simulink library "FVT_lib"  (R2021b)
settings: Solver=VariableStepAuto  StartTime=0.0  StopTime=10.0  RelTol=1e-3
undefined symbols (not defined in the file): C_TASK_5MS_S, CANFDArray, ENUM_FAULTSTATE_FAIL, ENUM_FAULTSTATE_INDETERMINATE, ENUM_FAULTSTATE_PASS, EPSILON, FALSE, KHAL_CounterMAX_enum, KHAL_CounterMAXE2E_enum, LINArray, ONE_INT, TRUE, UNKNOWN, XX2KXX, ZERO_FLOAT, ZERO_INT
libraries: hdlsllib x41, simulink x24, hcu_lib x7
(part 1 of 3)
settings Model: Creator=user  LastModifiedBy=FVT23010
settings SolverCC: AlgebraicLoopSolver=TrustRegion
settings DebuggingCC: SFMachineParentedDataDiag=warning

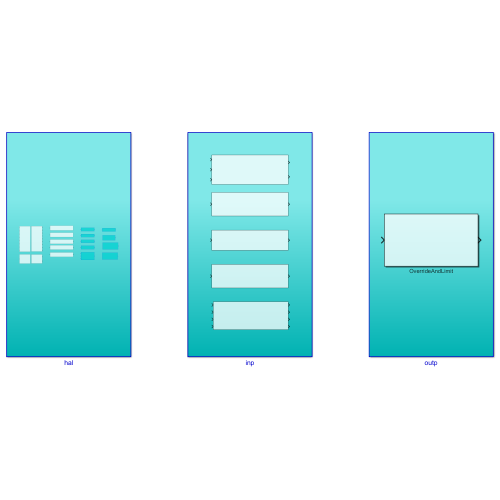
[thumbnail: Simulink's stored preview of the top-level diagram]
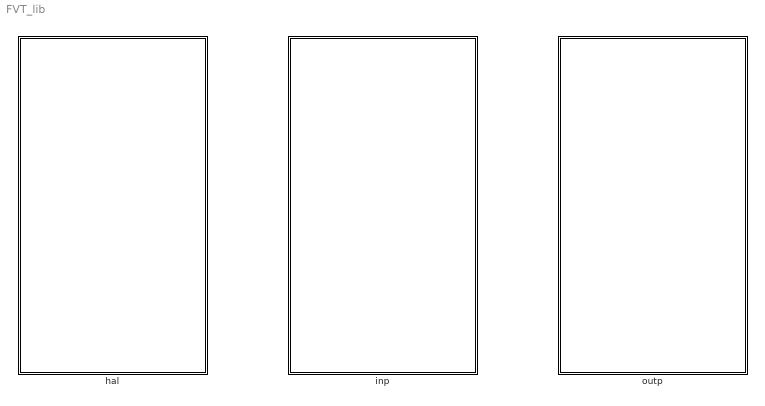
== system FVT_lib ==
  hal : Subsystem
  inp : Subsystem
  outp : Subsystem

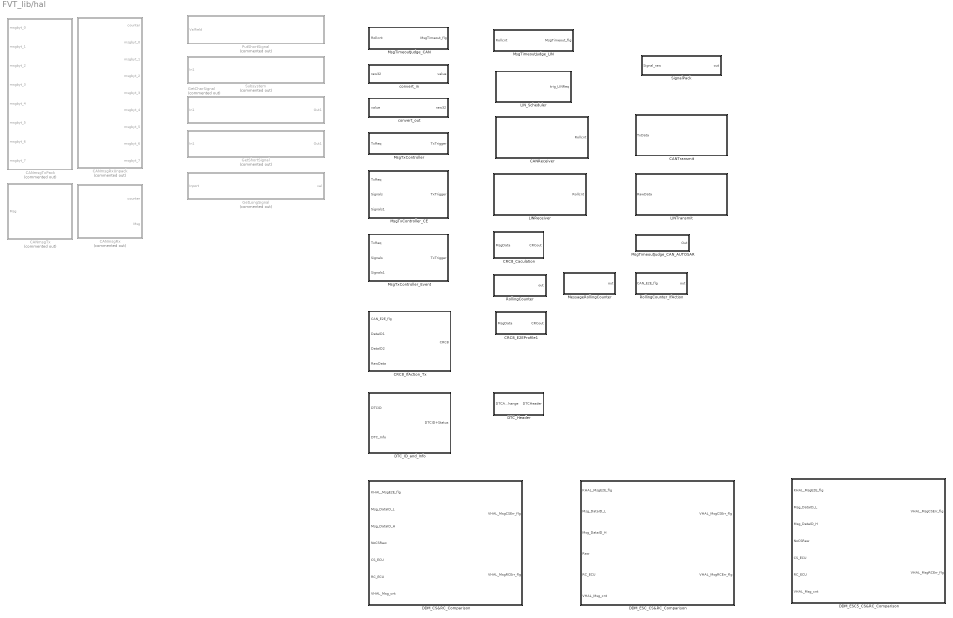
== system FVT_lib/hal ==
  CANReceiver : Subsystem  mask{busId=0, msgId=0x123, dlc=8}
      mask prompts: busId "BUS ID"; msgId "Message ID"
      mask Display:
      | fprintf('BUS ID: %1.0f \nMsg ID(hex): 0x%x \nDLC: %2.0f', busId, msgId,dlc);
      | 
      | port_label('output', 1, 'rolling counter');
  CANTransmit : Subsystem  mask{busId=0, msgId=0x123, dlc=8, IsCANFD=0}
      mask prompts: busId "BUS ID"; msgId "Message ID"
      mask Display:
      | fprintf('BUS ID: %1.0f \nMsg ID(hex): 0x%x \nDLC: %2.0f\nIs CANFD: %1.0f', busId, msgId,dlc,IsCANFD);
      | port_label('input', 1, 'Tx raw data');
  CANmsgRx : Subsystem  Commented=on  mask{rtwchn=CAN 1, rtwcode=367}
      mask prompts: rtwchn "Can channel :"; rtwcode "CAN ID :"
      mask TypeOptions rtwchn: CAN 1 | CAN 2 | CAN 3 | CAN 4
      mask Display:
      | fprintf('Receive Message on\nCAN %x \nID_hex: %x', rtwchn, rtwcode);
      | image('nxp_logo.png','top-left')
      | port_label('output', 1, 'rolling counter');
  CANmsgRxUnpack : Subsystem  Commented=on  mask{rtwchn=CAN 1, rtwcode=367}
      mask prompts: rtwchn "Can channel :"; rtwcode "CAN ID :"
      mask TypeOptions rtwchn: CAN 1 | CAN 2 | CAN 3 | CAN 4
      mask Display:
      | fprintf('Receive Message on\nCAN %x \nID_hex: %x', rtwchn, rtwcode);
      | image('nxp_logo.png','top-left')
      | port_label('output', 1, 'rolling counter');
  CANmsgTx : Subsystem  Commented=on  mask{rtwchn=CAN 1, rtwmrk=FALSE, rtwcode=367}
      mask prompts: rtwchn "Can channel :"; rtwmrk "Extend ID :"; rtwcode "CAN ID :"
      mask TypeOptions rtwchn: CAN 1 | CAN 2 | CAN 3 | CAN 4
      mask TypeOptions rtwmrk: FALSE | TRUE
      mask Display:
      | fprintf('Send Message on\nCAN %x \nID_hex: %x', rtwchn, rtwcode);
      | image('nxp_logo.png','top-left')
  CANmsgTxPack : Subsystem  Commented=on  mask{rtwchn=CAN 1, rtwmrk=FALSE, rtwcode=367}
      mask prompts: rtwchn "Can channel :"; rtwmrk "Extend ID :"; rtwcode "CAN ID :"
      mask TypeOptions rtwchn: CAN 1 | CAN 2 | CAN 3 | CAN 4
      mask TypeOptions rtwmrk: FALSE | TRUE
      mask Display:
      | fprintf('Send Message on\nCAN %x \nID_hex: %x', rtwchn, rtwcode);
      | image('nxp_logo.png','top-left')
  CRC8_Caculation : Subsystem
      mask help: MeasumentTrigerEvent
      mask Display: fprintf('CRC8');
  CRC8_E2EProfile1 : Subsystem
      mask help: MeasumentTrigerEvent
      mask Display: fprintf('CRC8_E2EProfile1');
  CRC8_IfAction_Tx : Subsystem
      mask help: MeasumentTrigerEvent
      mask Display: fprintf('CRC8_IfAction');
  DDM_CS&RC_Comparison : Subsystem  mask{MsgCycleTime=0}
      mask help: CS&RC Comparison
      mask Display:
      | fprintf('DDM_CS&RC_Comparison');
      | 
      | port_label('input', 1, 'KHAL_MsgE2E_flg');
      | port_label('input', 2, 'Msg_DataID_L');
      | port_label('input', 3, 'Msg_DataID_H');
      | port_label('input', 4, 'NoCSRaw');
      | port_label('input', 5, 'CS_ECU');
      | port_label('input', 6, 'RC_ECU');
      | port_label('input', 7, 'VHAL_Msg_cnt');
      | 
      | port_label('output', 1, 'VHAL_MsgCSErr_flg');
      | port_label('output', 2, 'VHAL_MsgRCErr_flg');
  DDM_ESC5_CS&RC_Comparison : Subsystem  mask{MsgCycleTime=0}
      mask help: CS&RC Comparison
      mask Display:
      | fprintf('DDM_ESC5_CS&RC_Comparison');
      | 
      | port_label('input', 1, 'KHAL_MsgE2E_flg');
      | port_label('input', 2, 'Msg_DataID_L');
      | port_label('input', 3, 'Msg_DataID_H');
      | port_label('input', 4, 'NoCSRaw');
      | port_label('input', 5, 'CS_ECU');
      | port_label('input', 6, 'RC_ECU');
      | port_label('input', 7, 'VHAL_Msg_cnt');
      | 
      | port_label('output', 1, 'VHAL_MsgCSErr_flg');
      | port_label('output', 2, 'VHAL_MsgRCErr_flg');
  DDM_ESC_CS&RC_Comparison : Subsystem  mask{MsgCycleTime=0}
      mask help: CS&RC Comparison
      mask Display:
      | fprintf('DDM_ESC_CS&RC_Comparison');
      | 
      | port_label('input', 1, 'KHAL_MsgE2E_flg');
      | port_label('input', 2, 'Msg_DataID_L');
      | port_label('input', 3, 'Msg_DataID_H');
      | port_label('input', 4, 'Raw');
      | port_label('input', 5, 'RC_ECU');
      | port_label('input', 6, 'VHAL_Msg_cnt');
      | 
      | port_label('output', 1, 'VHAL_MsgCSErr_flg');
      | port_label('output', 2, 'VHAL_MsgRCErr_flg');
  DTC_Header : Subsystem
      mask help: MeasumentTrigerEvent
      mask Display: fprintf('DTCHeader');
  DTC_ID_and_Info : Subsystem
      mask help: MeasumentTrigerEvent
      mask Display: fprintf('DTCID+Info');
  GetCharSignal : Subsystem  Commented=on  mask{CC1=55, CC2=8}
      mask prompts: CC1 "MSB:"; CC2 "DataLegth:"
      mask TypeOptions CC1: 0 | 1 | 2 | 3 | 4 | 5 | 6 | 7 | 8 | 9 | 10 | 11 | 12 | 13 | 14 | 15 | 16 | 17 | 18 | 19 | 20 | 21 | 22 | 23 | 24 | 25 | 26 | 27 | 28 | 29 | 30 | 31 | 32 | 33 | 34 | 35 | 36 | 37 | 38 | 39 | 40 | 41 | 42 | 43 | 44 | 45 | 46 | 47 | 48 | 49 | 50 | 51 | 52 | 53 | 54 | 55 | 56 | 57 | 58 | 59 | 60 | 61 | 62 | 63
      mask Display:
      | fprintf('Get Char Signal \nMSB: %d \nDLC: %d', CC1-1, CC2);
      | image('nxp_logo.png','top-left')
  GetLongSignal : Subsystem  Commented=on  mask{msb=0, len=0}
      mask prompts: len "Length"
      mask Display:
      | fprintf('Get Long Signal \nMSB: %d \nDLC: %d', msb, len);
      | image('nxp_logo.png','top-left')
  GetShortSignal : Subsystem  Commented=on  mask{CC1=23, CC2=12}
      mask prompts: CC1 "MSB:"; CC2 "DataLegth:"
      mask TypeOptions CC1: 0 | 1 | 2 | 3 | 4 | 5 | 6 | 7 | 8 | 9 | 10 | 11 | 12 | 13 | 14 | 15 | 16 | 17 | 18 | 19 | 20 | 21 | 22 | 23 | 24 | 25 | 26 | 27 | 28 | 29 | 30 | 31 | 32 | 33 | 34 | 35 | 36 | 37 | 38 | 39 | 40 | 41 | 42 | 43 | 44 | 45 | 46 | 47 | 48 | 49 | 50 | 51 | 52 | 53 | 54 | 55 | 56 | 57 | 58 | 59 | 60 | 61 | 62 | 63
      mask Display:
      | fprintf('Get Short Signal \nMSB: %d \nDLC: %d', CC1-1, CC2);
      | image('nxp_logo.png','top-left')
  LINReceiver : Subsystem  mask{busId=0, msgId=0x123, dlc=8}
      mask prompts: busId "BUS ID"; msgId "Message ID"
      mask Display:
      | fprintf('BUS ID: %1.0f \nMsg ID(hex): 0x%x \nDLC: %2.0f', busId, msgId,dlc);
      | port_label('output', 1, 'fault counter');
  LINTransmit : Subsystem  mask{busId=0, msgId=0x123, dlc=8}
      mask prompts: busId "BUS ID"; msgId "Message ID"
      mask Display:
      | fprintf('BUS ID: %1.0f \nMsg ID(hex): 0x%x \nDLC: %2.0f', busId, msgId,dlc);
      | port_label('input', 1, 'Tx raw data');
  LIN_Scheduler : Subsystem  mask{CycleTime=100, FirstDelayTime=80}
      mask prompts: CycleTime "CycleTime_ms"; FirstDelayTime "DelayTime_ms"
      mask Display: fprintf('Total cycle time(ms): %d\nFirst delay time(ms): %3.0f', CycleTime, FirstDelayTime);
  MessageRollingCounter : Subsystem  mask{CounterMAX=14, task_time_ms=5, msg_time_ms=10}
      mask help: MeasumentTrigerEvent
      mask Display: fprintf('MsgRC');
  MsgTimeoutJudge_CAN : Subsystem  mask{Gain=1.5, CycleTime=100}
      mask prompts: CycleTime "MsgCycleTime_ms"
      mask help: MeasumentTrigerTime
      mask Display: fprintf('Gain: %4.2f \nMsg Cycletime ms: %3.0f', Gain, CycleTime);
  MsgTimeoutJudge_CAN_AUTOSAR : Subsystem
      mask help: MeasumentTrigerEvent
      mask Display: fprintf('MsgTimeoutJudge_CAN\nAUTOSAR');
  MsgTimeoutJudge_LIN : Subsystem  mask{TimeoutCnt=3}
      mask help: MeasumentTrigerTime
      mask Display: fprintf('TimeoutCnt: %4.2f', TimeoutCnt);
  MsgTxController : Subsystem  mask{CycleTime=100}
      mask prompts: CycleTime "MsgCycleTime_ms"
      mask help: MeasumentTrigerTime
      mask Display: fprintf('Tx Method: Cycle\nMsg Cycletime ms: %3.0f', CycleTime);
  MsgTxController_CE : Subsystem  mask{CycleTime=100}
      mask prompts: CycleTime "MsgCycleTime_ms"
      mask help: MeasumentTrigerTime
      mask Display: fprintf('Tx Method: CE\nMsg Cycletime ms: %3.0f', CycleTime);
  MsgTxController_Event : Subsystem
      mask help: MeasumentTrigerEvent
      mask Display: fprintf('Tx Method: Event');
  PutShortSignal : Subsystem  Commented=on  mask{SS1=5, SS2=13, SS3=[0 0 0 0 0 0 0 0]}
      mask prompts: SS1 "MSB:"; SS2 "DataLeght:"; SS3 "MsgBuffer:"
      mask TypeOptions SS1: 0 | 1 | 2 | 3 | 4 | 5 | 6 | 7 | 8 | 9 | 10 | 11 | 12 | 13 | 14 | 15 | 16 | 17 | 18 | 19 | 20 | 21 | 22 | 23 | 24 | 25 | 26 | 27 | 28 | 29 | 30 | 31 | 32 | 33 | 34 | 35 | 36 | 37 | 38 | 39 | 40 | 41 | 42 | 43 | 44 | 45 | 46 | 47 | 48 | 49 | 50 | 51 | 52 | 53 | 54 | 55 | 56 | 57 | 58 | 59 | 60 | 61 | 62 | 63
      mask Display:
      | fprintf('Put Short Signal \nMSB: %d \nDLC: %d', SS1-1, SS2);
      | image('nxp_logo.png','top-left')
  RollingCounter : Subsystem  mask{CounterMAX=14}
      mask help: MeasumentTrigerEvent
      mask Display: fprintf('RollingCounter');
  RollingCounter_IfAction : Subsystem
      mask help: MeasumentTrigerEvent
      mask Display: fprintf('RollingCounter_IfAction');
  SignalPack : Subsystem  mask(ConvertOut){RightShiftCnt=0, BitMask=2^1-1, LeftShiftCnt=0}
      mask prompts: BitMask "Bit mask"
      mask help:
      | Conversion Formula
      |
      | The conversion formula is
      |
      | raw_value = (physical_value - Offset) / Factor
      |
      | where physical_value is the value of the signal after it is saturated using the specified Min and Max values. raw_value is the packed signal value.
      mask Display: fprintf('RightShiftCnt: %1.0f \nMASK: %d \nLeftShiftCnt: %1.0f', RightShiftCnt, BitMask, LeftShiftCnt);
  Subsystem : Subsystem  Commented=on  mask{SS1=47, SS2=8, SS3=[0 0 0 0 0 0 0 0]}
      mask prompts: SS1 "MSB:"; SS2 "DataLegth:"; SS3 "MsgBuffer:"
      mask TypeOptions SS1: 0 | 1 | 2 | 3 | 4 | 5 | 6 | 7 | 8 | 9 | 10 | 11 | 12 | 13 | 14 | 15 | 16 | 17 | 18 | 19 | 20 | 21 | 22 | 23 | 24 | 25 | 26 | 27 | 28 | 29 | 30 | 31 | 32 | 33 | 34 | 35 | 36 | 37 | 38 | 39 | 40 | 41 | 42 | 43 | 44 | 45 | 46 | 47 | 48 | 49 | 50 | 51 | 52 | 53 | 54 | 55 | 56 | 57 | 58 | 59 | 60 | 61 | 62 | 63
      mask Display:
      | fprintf('Put Char Signal \nMSB: %d \nDLC: %d', SS1-1, SS2);
      | image('nxp_logo.png','top-left')
  convert_in : Subsystem  mask(ConvertIn){gain=1, offset=1}
      mask help:
      | Conversion Formula
      |
      | The conversion formula is
      |
      | raw_value = (physical_value - Offset) / Factor
      |
      | where physical_value is the value of the signal after it is saturated using the specified Min and Max values. raw_value is the packed signal value.
      mask Display: fprintf('Resolution: %6.4f \nOffset: %5.0f', gain, offset);
  convert_out : Subsystem  mask(ConvertOut){gain=1, offset=1}
      mask help:
      | Conversion Formula
      |
      | The conversion formula is
      |
      | raw_value = (physical_value - Offset) / Factor
      |
      | where physical_value is the value of the signal after it is saturated using the specified Min and Max values. raw_value is the packed signal value.
      mask Display: fprintf('Resolution: %6.4f \nOffset: %5.0f', gain, offset);

== system FVT_lib/inp ==
  CAN_Msg_Validity_Process_template : Subsystem
  ad_signal_template : Subsystem
  can_signal_template : Subsystem
      settings: RTWSystemCode=Inline
  di_signal_template : Subsystem
  pwm_signal_template : Subsystem

== system FVT_lib/outp ==
  OverrideAndLimit : Subsystem

== system FVT_lib/hal/CANReceiver ==
  CANReceive : CCaller  FunctionName=CANReceive  PortSpecificationStruct="%)30     .    T @   8    (     @         %    \"     4    !     0         %  0 \"0    $    _    07)G3F%M90  4&]R=$YA;64 4V-O<&4     26YD97@     5'EP90      4VEZ90      27-';&]B86P   X    P    !@    @    $          4    (     0    ,    !         !   P!O=70 #@   #     &    \"     0         !0    @    !     P    $         $  # &]U=  .    .     8    (    !          %    \"     $    &     0         0   ...(+2654 chars)"
  Constant6 : Constant  Value=busId
  Constant7 : Constant  Value=CANFDArray
  Constant8 : Constant  Value=msgId
  Constant9 : Constant  Value=dlc
  Data Type Conversion16 : DataTypeConversion  OutDataTypeStr=uint8
  Data Type Conversion17 : DataTypeConversion  OutDataTypeStr=uint16
  Data Type Conversion18 : DataTypeConversion  OutDataTypeStr=uint8
  Data Type Conversion19 : DataTypeConversion  OutDataTypeStr=uint8
  Demux : Demux  Outputs=16
  Rollcnt : Outport
  wires:
  Data Type Conversion19/1 -> CANReceive/3
  Constant8/1 -> Data Type Conversion17/1
  Constant6/1 -> Data Type Conversion16/1
  Constant9/1 -> Data Type Conversion18/1
  Data Type Conversion17/1 -> CANReceive/2
  Data Type Conversion16/1 -> CANReceive/1
  Data Type Conversion18/1 -> CANReceive/4
  Constant7/1 -> Data Type Conversion19/1
  [RxData] -> Demux/1
  CANReceive/2 -> [RxData]
  CANReceive/1 -> Rollcnt/1

== system FVT_lib/hal/CANTransmit ==
  TxData : Inport
  C Caller : CCaller  FunctionName=CANTransmit  PortSpecificationStruct="%)30     .    R @   8    (     @         %    \"     4    !     0         %  0 \"0    $    _    07)G3F%M90  4&]R=$YA;64 4V-O<&4     26YD97@     5'EP90      4VEZ90      27-';&]B86P   X    X    !@    @    $          4    (     0    4    !         !     %    8G5S260    .    .     8    (    !          %    \"     $    %     0         0    !0   &)U<TED    #@   #@    &    \"     0         !0    @    !   ...(+2646 chars)"
  Constant2 : Constant  Value=busId
  Constant3 : Constant  Value=msgId
  Constant4 : Constant  Value=IsCANFD
  Constant5 : Constant  Value=dlc
  UnitConverter5 : DataTypeConversion  OutDataTypeStr=uint8
  UnitConverter6 : DataTypeConversion  OutDataTypeStr=uint16
  UnitConverter7 : DataTypeConversion  OutDataTypeStr=uint8
  UnitConverter8 : DataTypeConversion  OutDataTypeStr=uint8
  wires:
  UnitConverter7/1 -> C Caller/3
  UnitConverter6/1 -> C Caller/2
  UnitConverter5/1 -> C Caller/1
  Constant5/1 -> UnitConverter8/1
  Constant3/1 -> UnitConverter6/1
  Constant4/1 -> UnitConverter7/1
  Constant2/1 -> UnitConverter5/1
  UnitConverter8/1 -> C Caller/5
  TxData/1 -> C Caller/4

== system FVT_lib/hal/CANmsgRx ==
  Constant : Constant  Value=rtwcode  OutDataTypeStr=uint32
  Data Type Conversion7 : DataTypeConversion  OutDataTypeStr=uint8
  sfcnCanLLGetMessage : S-Function  FunctionName=sfcnCanLLGetMessage  Parameters=SParameter1  SFunctionDeploymentMode=off  EnableBusSupport=off  mask{SParameter1=rtwchn-1}
      mask prompts: SParameter1 "P1:"
      mask Display: fprintf('Level-2 S-Function CanLLGetMessage');
  counter : Outport
  Msg : Outport  Port=2
  wires:
  Data Type Conversion7/1 -> counter/1
  sfcnCanLLGetMessage/1 -> Data Type Conversion7/1
  Constant/1 -> sfcnCanLLGetMessage/1
  sfcnCanLLGetMessage/2 -> Msg/1

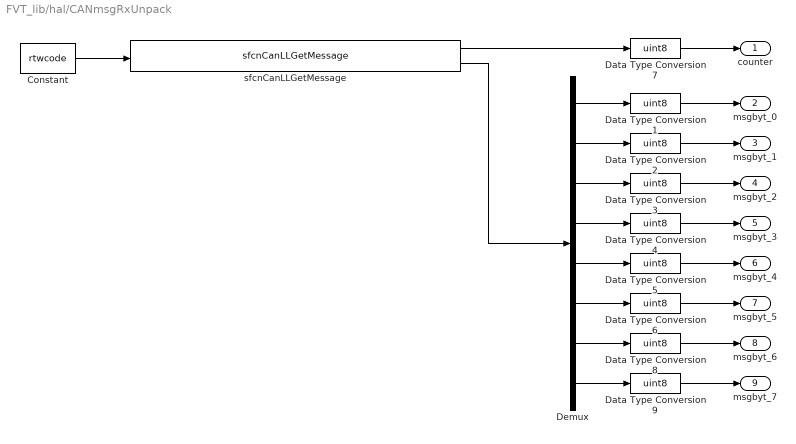
== system FVT_lib/hal/CANmsgRxUnpack ==
  Constant : Constant  Value=rtwcode  OutDataTypeStr=uint32
  Data Type Conversion{1..9} (9 alike) : DataTypeConversion  OutDataTypeStr=uint8
  Demux : Demux  Outputs=8
  sfcnCanLLGetMessage : S-Function  FunctionName=sfcnCanLLGetMessage  Parameters=SParameter1  SFunctionDeploymentMode=off  EnableBusSupport=off  mask{SParameter1=rtwchn-1}
      mask prompts: SParameter1 "P1:"
      mask Display: fprintf('Level-2 S-Function CanLLGetMessage');
  counter : Outport
  msgbyt_0 : Outport  Port=2
  msgbyt_1 : Outport  Port=3
  msgbyt_2 : Outport  Port=4
  msgbyt_3 : Outport  Port=5
  msgbyt_4 : Outport  Port=6
  msgbyt_5 : Outport  Port=7
  msgbyt_6 : Outport  Port=8
  msgbyt_7 : Outport  Port=9
  wires:
  Demux/1 -> Data Type Conversion1/1
  Demux/4 -> Data Type Conversion4/1
  Constant/1 -> sfcnCanLLGetMessage/1
  Demux/6 -> Data Type Conversion6/1
  Demux/3 -> Data Type Conversion3/1
  Demux/8 -> Data Type Conversion9/1
  Demux/2 -> Data Type Conversion2/1
  Demux/5 -> Data Type Conversion5/1
  Demux/7 -> Data Type Conversion8/1
  sfcnCanLLGetMessage/1 -> Data Type Conversion7/1
  sfcnCanLLGetMessage/2 -> Demux/1
  Data Type Conversion7/1 -> counter/1
  Data Type Conversion1/1 -> msgbyt_0/1
  Data Type Conversion2/1 -> msgbyt_1/1
  Data Type Conversion4/1 -> msgbyt_3/1
  Data Type Conversion3/1 -> msgbyt_2/1
  Data Type Conversion5/1 -> msgbyt_4/1
  Data Type Conversion8/1 -> msgbyt_6/1
  Data Type Conversion6/1 -> msgbyt_5/1
  Data Type Conversion9/1 -> msgbyt_7/1

== system FVT_lib/hal/CANmsgTx ==
  Msg : Inport
  Constant4 : Constant  Value=rtwcode  OutDataTypeStr=uint32
  Constant6 : Constant  Value=rtwmrk-1  OutDataTypeStr=uint8
  Data Type Conversion : DataTypeConversion  OutDataTypeStr=uint8
  sfcnCanLLSendMessage : S-Function  FunctionName=sfcnCanLLSendMessage  Parameters=SParameter1  SFunctionDeploymentMode=off  EnableBusSupport=off  mask{SParameter1=rtwchn-1}
      mask prompts: SParameter1 "P1:"
      mask Display: fprintf('Level-2 S-Function CanLLSendMessage');
  wires:
  Data Type Conversion/1 -> sfcnCanLLSendMessage/3
  Msg/1 -> Data Type Conversion/1
  Constant4/1 -> sfcnCanLLSendMessage/1
  Constant6/1 -> sfcnCanLLSendMessage/2

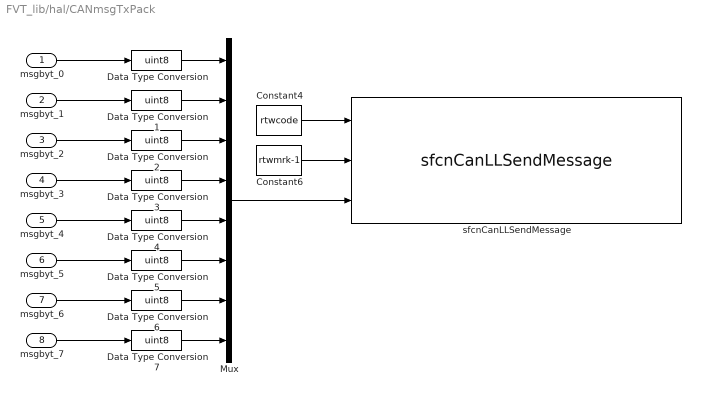
== system FVT_lib/hal/CANmsgTxPack ==
  msgbyt_0 : Inport
  msgbyt_1 : Inport  Port=2
  msgbyt_2 : Inport  Port=3
  msgbyt_3 : Inport  Port=4
  msgbyt_4 : Inport  Port=5
  msgbyt_5 : Inport  Port=6
  msgbyt_6 : Inport  Port=7
  msgbyt_7 : Inport  Port=8
  Constant4 : Constant  Value=rtwcode  OutDataTypeStr=uint32
  Constant6 : Constant  Value=rtwmrk-1  OutDataTypeStr=uint8
  Data Type Conversion{,1..7} (8 alike) : DataTypeConversion  OutDataTypeStr=uint8
  Mux : Mux  Inputs=8
  sfcnCanLLSendMessage : S-Function  FunctionName=sfcnCanLLSendMessage  Parameters=SParameter1  SFunctionDeploymentMode=off  EnableBusSupport=off  mask{SParameter1=rtwchn-1}
      mask prompts: SParameter1 "P1:"
      mask Display: fprintf('Level-2 S-Function CanLLSendMessage');
  wires:
  Constant6/1 -> sfcnCanLLSendMessage/2
  Constant4/1 -> sfcnCanLLSendMessage/1
  msgbyt_1/1 -> Data Type Conversion1/1
  msgbyt_3/1 -> Data Type Conversion3/1
  msgbyt_6/1 -> Data Type Conversion6/1
  msgbyt_5/1 -> Data Type Conversion5/1
  msgbyt_0/1 -> Data Type Conversion/1
  msgbyt_7/1 -> Data Type Conversion7/1
  msgbyt_4/1 -> Data Type Conversion4/1
  msgbyt_2/1 -> Data Type Conversion2/1
  Mux/1 -> sfcnCanLLSendMessage/3
  Data Type Conversion/1 -> Mux/1
  Data Type Conversion1/1 -> Mux/2
  Data Type Conversion2/1 -> Mux/3
  Data Type Conversion3/1 -> Mux/4
  Data Type Conversion4/1 -> Mux/5
  Data Type Conversion5/1 -> Mux/6
  Data Type Conversion6/1 -> Mux/7
  Data Type Conversion7/1 -> Mux/8

== system FVT_lib/hal/CRC8_Caculation ==
  MsgData : Inport
  Data Type Conversion3 : DataTypeConversion  OutDataTypeStr=uint8
  Data Type Conversion4 : DataTypeConversion  OutDataTypeStr=uint8
  MATLAB Function : MATLAB Function  TreatAsAtomicUnit=on
  CRCout : Outport
  wires:
  Data Type Conversion4/1 -> CRCout/1
  MATLAB Function/1(CRC_Out) -> Data Type Conversion4/1
  Data Type Conversion3/1 -> MATLAB Function/1(msg_raw)
  MsgData/1 -> Data Type Conversion3/1

== system FVT_lib/hal/CRC8_E2EProfile1 ==
  MsgData : Inport
  Data Type Conversion3 : DataTypeConversion  OutDataTypeStr=uint8
  Data Type Conversion4 : DataTypeConversion  OutDataTypeStr=uint8
  MATLAB Function : MATLAB Function  TreatAsAtomicUnit=on
  CRCout : Outport
  wires:
  MsgData/1 -> Data Type Conversion3/1
  Data Type Conversion3/1 -> MATLAB Function/1(msg_raw)
  MATLAB Function/1(CRC_Out) -> Data Type Conversion4/1
  Data Type Conversion4/1 -> CRCout/1

== system FVT_lib/hal/CRC8_IfAction_Tx ==
  CAN_E2E_flg : Inport
  DataID1 : Inport  Port=2
  DataID2 : Inport  Port=3
  RawData : Inport  Port=4
  Data Type Conversion : DataTypeConversion  OutDataTypeStr=uint8
  If : If
  If Action Subsystem : Subsystem  TreatAsAtomicUnit=on
  If Action Subsystem1 : Subsystem  TreatAsAtomicUnit=on
  Merge : Merge
  CRC8 : Outport
  wires:
  Data Type Conversion/1 -> If/1
  Merge/1 -> CRC8/1
  If Action Subsystem/1(CRC8_Result) -> Merge/2
  If Action Subsystem1/1(CRC8_E2EResult) -> Merge/1
  [RawData] -> If Action Subsystem/1(Byte1)
  [RawData] -> If Action Subsystem1/3(Byte1)
  [DataID2] -> If Action Subsystem1/2(CAN_E2E_ID2)
  [DataID1] -> If Action Subsystem1/1(CAN_E2E_ID1)
  [CAN_E2E_flg] -> Data Type Conversion/1
  RawData/1 -> [RawData]
  DataID2/1 -> [DataID2]
  DataID1/1 -> [DataID1]
  CAN_E2E_flg/1 -> [CAN_E2E_flg]
  If/1 -> If Action Subsystem1/Action
  If/2 -> If Action Subsystem/Action

== system FVT_lib/hal/DDM_CS&RC_Comparison ==
  KHAL_MsgE2E_flg : Inport
  Msg_DataID_L : Inport  Port=2
  Msg_DataID_H : Inport  Port=3
  NoCSRaw : Inport  Port=4
  CS_ECU : Inport  Port=5
  RC_ECU : Inport  Port=6
  VHAL_Msg_cnt : Inport  Port=7
  CRC8_Compare : Subsystem  mask{MissingNumLimit=2, RepeatNumLimit=1, CounterMAX=15, CounterMAX_E2E=14}
      mask help: MeasumentTrigerEvent
      mask Display: fprintf('CS & RC_Compare');
  CRC8_IfAction_Rx : Subsystem
      mask help: MeasumentTrigerEvent
      mask Display: fprintf('CRC8_IfAction');
  Constant5 : Constant  Value=MsgCycleTime  OutDataTypeStr=single
  Gain : Gain  Gain=1.5
  Gain1 : Gain  Gain=XX2KXX
  VHAL_MsgCSErr_flg : Outport
  VHAL_MsgRCErr_flg : Outport  Port=2
  wires:
  Msg_DataID_H/1 -> CRC8_IfAction_Rx/3(CAN_E2E_ID2)
  Msg_DataID_L/1 -> CRC8_IfAction_Rx/2(CAN_E2E_ID1)
  KHAL_MsgE2E_flg/1 -> CRC8_Compare/5(CAN_E2E_flg), CRC8_IfAction_Rx/1(CAN_E2E_flg)
  CRC8_Compare/1(CS_Error) -> VHAL_MsgCSErr_flg/1
  CRC8_Compare/2(RC_Error) -> VHAL_MsgRCErr_flg/1
  CS_ECU/1 -> CRC8_Compare/1(MsgData)
  NoCSRaw/1 -> CRC8_Compare/6(noCSRaw), CRC8_IfAction_Rx/4(Raw)
  RC_ECU/1 -> CRC8_Compare/3(RC)
  VHAL_Msg_cnt/1 -> CRC8_Compare/4(MsgCnt)
  CRC8_IfAction_Rx/1(CRC8) -> CRC8_Compare/2(CRC8_Data)
  Gain/1 -> CRC8_Compare/7(RepeatTimeLimit)
  Constant5/1 -> Gain1/1
  Gain1/1 -> Gain/1

== system FVT_lib/hal/DDM_ESC5_CS&RC_Comparison ==
  KHAL_MsgE2E_flg : Inport
  Msg_DataID_L : Inport  Port=2
  Msg_DataID_H : Inport  Port=3
  NoCSRaw : Inport  Port=4
  CS_ECU : Inport  Port=5
  RC_ECU : Inport  Port=6
  VHAL_Msg_cnt : Inport  Port=7
  CRC8_Compare : Subsystem  mask{MissingNumLimit=2, RepeatNumLimit=1, CounterMAX=15, CounterMAX_E2E=14}
      mask help: MeasumentTrigerEvent
      mask Display: fprintf('CS & RC_Compare');
  CRC8_IfAction_Rx : Subsystem
      mask help: MeasumentTrigerEvent
      mask Display: fprintf('CRC8_IfAction');
  Constant5 : Constant  Value=MsgCycleTime  OutDataTypeStr=single
  Gain : Gain  Gain=1.5
  Gain1 : Gain  Gain=XX2KXX
  VHAL_MsgCSErr_flg : Outport
  VHAL_MsgRCErr_flg : Outport  Port=2
  wires:
  CRC8_IfAction_Rx/1(CRC8) -> CRC8_Compare/2(CRC8_Data)
  VHAL_Msg_cnt/1 -> CRC8_Compare/4(MsgCnt)
  RC_ECU/1 -> CRC8_Compare/3(RC)
  NoCSRaw/1 -> CRC8_Compare/6(noCSRaw), CRC8_IfAction_Rx/4(Raw)
  CS_ECU/1 -> CRC8_Compare/1(MsgData)
  CRC8_Compare/2(RC_Error) -> VHAL_MsgRCErr_flg/1
  CRC8_Compare/1(CS_Error) -> VHAL_MsgCSErr_flg/1
  KHAL_MsgE2E_flg/1 -> CRC8_IfAction_Rx/1(CAN_E2E_flg), CRC8_Compare/5(CAN_E2E_flg)
  Msg_DataID_L/1 -> CRC8_IfAction_Rx/2(CAN_E2E_ID1)
  Msg_DataID_H/1 -> CRC8_IfAction_Rx/3(CAN_E2E_ID2)
  Constant5/1 -> Gain1/1
  Gain/1 -> CRC8_Compare/7(RepeatTimeLimit)
  Gain1/1 -> Gain/1

== system FVT_lib/hal/DDM_ESC_CS&RC_Comparison ==
  KHAL_MsgE2E_flg : Inport
  Msg_DataID_L : Inport  Port=2
  Msg_DataID_H : Inport  Port=3
  Raw : Inport  Port=4
  RC_ECU : Inport  Port=5
  VHAL_Msg_cnt : Inport  Port=6
  Constant5 : Constant  Value=MsgCycleTime  OutDataTypeStr=single
  Demux : Demux  Outputs=8
  ESC_CS_Comparison : Subsystem
      mask help: ESC CS Comparison
      mask Display:
      | fprintf('ESC_CS_Comparison');
      | 
      | port_label('input', 1, 'Byte0');
      | port_label('input', 2, 'Byte1');
      | port_label('input', 3, 'Byte2');
      | port_label('input', 4, 'Byte3');
      | port_label('input', 5, 'Byte4');
      | port_label('input', 6, 'Byte5');
      | port_label('input', 7, 'Byte6');
      | port_label('input', 8, 'Byte7');
      | 
      | port_label('output', 1, 'CS_Equal_flg');
  Gain : Gain  Gain=1.5
  Gain1 : Gain  Gain=XX2KXX
  Logical Operator : Logic  Operator=NOT  AllPortsSameDT=off  OutDataTypeStr=boolean
  RC_Compare : Subsystem  mask{MissingNumLimit=2, RepeatNumLimit=1, CounterMAX=15, CounterMAX_E2E=14}
      mask help: MeasumentTrigerEvent
      mask Display: fprintf('RC_Compare');
  Terminator : Terminator
  Terminator1 : Terminator
  VHAL_MsgCSErr_flg : Outport
  VHAL_MsgRCErr_flg : Outport  Port=2
  wires:
  VHAL_Msg_cnt/1 -> RC_Compare/2(MsgCnt)
  RC_ECU/1 -> RC_Compare/1(RC)
  RC_Compare/1(RC_Error) -> VHAL_MsgRCErr_flg/1
  ESC_CS_Comparison/1(CS_Equal_flg) -> Logical Operator/1
  Logical Operator/1 -> VHAL_MsgCSErr_flg/1
  KHAL_MsgE2E_flg/1 -> RC_Compare/3(CAN_E2E_flg)
  Demux/1 -> ESC_CS_Comparison/1(byte0)
  Demux/2 -> ESC_CS_Comparison/2(byte1)
  Demux/3 -> ESC_CS_Comparison/3(byte2)
  Demux/4 -> ESC_CS_Comparison/4(byte3)
  Demux/5 -> ESC_CS_Comparison/5(byte4)
  Demux/6 -> ESC_CS_Comparison/6(byte5)
  Demux/7 -> ESC_CS_Comparison/7(byte6)
  Demux/8 -> ESC_CS_Comparison/8(byte7)
  Raw/1 -> RC_Compare/4(noCSRaw), Demux/1
  Msg_DataID_L/1 -> Terminator/1
  Msg_DataID_H/1 -> Terminator1/1
  Constant5/1 -> Gain1/1
  Gain/1 -> RC_Compare/5(RepeatTimeLimit)
  Gain1/1 -> Gain/1

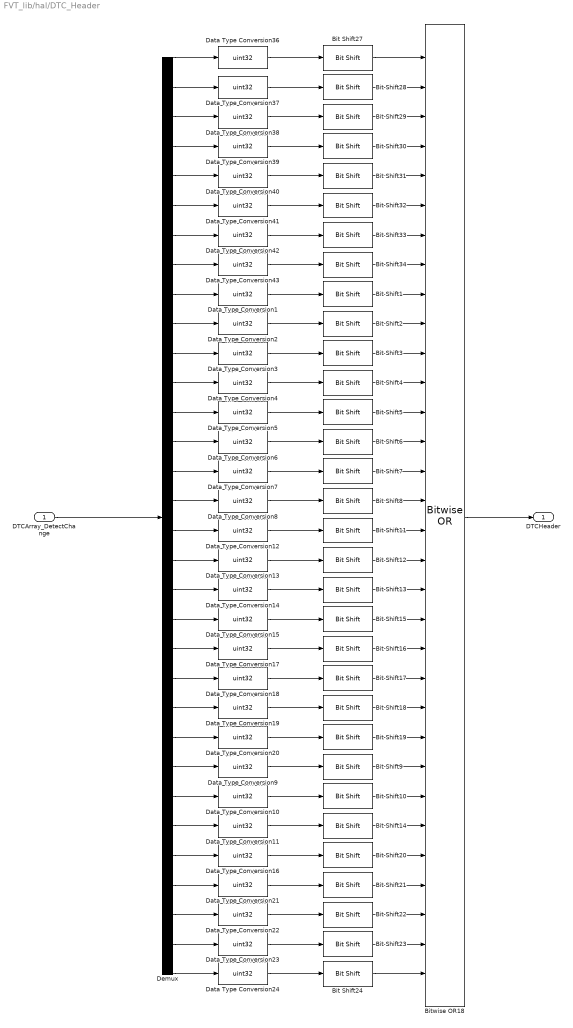
== system FVT_lib/hal/DTC_Header ==
  DTCArray_DetectChange : Inport
  Bit Shift1 : hdlsllib/Logic and Bit Operations/Bit Shift  mode=Shift Left Logical  N=23
  Bit Shift10 : hdlsllib/Logic and Bit Operations/Bit Shift  mode=Shift Left Logical  N=6
  Bit Shift11 : hdlsllib/Logic and Bit Operations/Bit Shift  mode=Shift Left Logical  N=15
  Bit Shift12 : hdlsllib/Logic and Bit Operations/Bit Shift  mode=Shift Left Logical  N=14
  Bit Shift13 : hdlsllib/Logic and Bit Operations/Bit Shift  mode=Shift Left Logical  N=13
  Bit Shift14 : hdlsllib/Logic and Bit Operations/Bit Shift  mode=Shift Left Logical  N=5
  Bit Shift15 : hdlsllib/Logic and Bit Operations/Bit Shift  mode=Shift Left Logical  N=12
  Bit Shift16 : hdlsllib/Logic and Bit Operations/Bit Shift  mode=Shift Left Logical  N=11
  Bit Shift17 : hdlsllib/Logic and Bit Operations/Bit Shift  mode=Shift Left Logical  N=10
  Bit Shift18 : hdlsllib/Logic and Bit Operations/Bit Shift  mode=Shift Left Logical  N=9
  Bit Shift19 : hdlsllib/Logic and Bit Operations/Bit Shift  mode=Shift Left Logical  N=8
  Bit Shift2 : hdlsllib/Logic and Bit Operations/Bit Shift  mode=Shift Left Logical  N=22
  Bit Shift20 : hdlsllib/Logic and Bit Operations/Bit Shift  mode=Shift Left Logical  N=4
  Bit Shift21 : hdlsllib/Logic and Bit Operations/Bit Shift  mode=Shift Left Logical  N=3
  Bit Shift22 : hdlsllib/Logic and Bit Operations/Bit Shift  mode=Shift Left Logical  N=2
  Bit Shift23 : hdlsllib/Logic and Bit Operations/Bit Shift  mode=Shift Left Logical  N=1
  Bit Shift24 : hdlsllib/Logic and Bit Operations/Bit Shift  mode=Shift Left Logical  N=0
  Bit Shift27 : hdlsllib/Logic and Bit Operations/Bit Shift  mode=Shift Left Logical  N=31
  Bit Shift28 : hdlsllib/Logic and Bit Operations/Bit Shift  mode=Shift Left Logical  N=30
  Bit Shift29 : hdlsllib/Logic and Bit Operations/Bit Shift  mode=Shift Left Logical  N=29
  Bit Shift3 : hdlsllib/Logic and Bit Operations/Bit Shift  mode=Shift Left Logical  N=21
  Bit Shift30 : hdlsllib/Logic and Bit Operations/Bit Shift  mode=Shift Left Logical  N=28
  Bit Shift31 : hdlsllib/Logic and Bit Operations/Bit Shift  mode=Shift Left Logical  N=27
  Bit Shift32 : hdlsllib/Logic and Bit Operations/Bit Shift  mode=Shift Left Logical  N=26
  Bit Shift33 : hdlsllib/Logic and Bit Operations/Bit Shift  mode=Shift Left Logical  N=25
  Bit Shift34 : hdlsllib/Logic and Bit Operations/Bit Shift  mode=Shift Left Logical  N=24
  Bit Shift4 : hdlsllib/Logic and Bit Operations/Bit Shift  mode=Shift Left Logical  N=20
  Bit Shift5 : hdlsllib/Logic and Bit Operations/Bit Shift  mode=Shift Left Logical  N=19
  Bit Shift6 : hdlsllib/Logic and Bit Operations/Bit Shift  mode=Shift Left Logical  N=18
  Bit Shift7 : hdlsllib/Logic and Bit Operations/Bit Shift  mode=Shift Left Logical  N=17
  Bit Shift8 : hdlsllib/Logic and Bit Operations/Bit Shift  mode=Shift Left Logical  N=16
  Bit Shift9 : hdlsllib/Logic and Bit Operations/Bit Shift  mode=Shift Left Logical  N=7
  Bitwise OR18 : simulink/Logic and Bit Operations/Bitwise Operator  logicop=OR  UseBitMask=off  NumInputPorts=32  BitMask=bin2dec('11011001')  BitMaskRealWorld=Stored Integer
  Data Type Conversion{1..24,36..43} (32 alike) : DataTypeConversion  OutDataTypeStr=uint32
  Demux : Demux  Outputs=32
  DTCHeader : Outport
  wires:
  Bit Shift23/1 -> Bitwise OR18/31
  Demux/6 -> Data Type Conversion41/1
  Demux/4 -> Data Type Conversion39/1
  Bit Shift28/1 -> Bitwise OR18/2
  Demux/1 -> Data Type Conversion36/1
  Data Type Conversion41/1 -> Bit Shift32/1
  Demux/16 -> Data Type Conversion8/1
  Data Type Conversion14/1 -> Bit Shift13/1
  Data Type Conversion42/1 -> Bit Shift33/1
  Demux/31 -> Data Type Conversion23/1
  Demux/15 -> Data Type Conversion7/1
  Data Type Conversion43/1 -> Bit Shift34/1
  Data Type Conversion21/1 -> Bit Shift21/1
  Bit Shift31/1 -> Bitwise OR18/5
  Demux/28 -> Data Type Conversion16/1
  Bit Shift13/1 -> Bitwise OR18/19
  Bit Shift14/1 -> Bitwise OR18/27
  Demux/17 -> Data Type Conversion12/1
  Data Type Conversion23/1 -> Bit Shift23/1
  Bit Shift32/1 -> Bitwise OR18/6
  Bit Shift5/1 -> Bitwise OR18/13
  Demux/12 -> Data Type Conversion4/1
  Bit Shift2/1 -> Bitwise OR18/10
  Bit Shift29/1 -> Bitwise OR18/3
  Bit Shift1/1 -> Bitwise OR18/9
  Bit Shift12/1 -> Bitwise OR18/18
  Data Type Conversion10/1 -> Bit Shift10/1
  Data Type Conversion22/1 -> Bit Shift22/1
  Bit Shift24/1 -> Bitwise OR18/32
  Data Type Conversion5/1 -> Bit Shift5/1
  Bit Shift22/1 -> Bitwise OR18/30
  Data Type Conversion9/1 -> Bit Shift9/1
  Data Type Conversion12/1 -> Bit Shift11/1
  Data Type Conversion4/1 -> Bit Shift4/1
  Bit Shift18/1 -> Bitwise OR18/23
  Bit Shift21/1 -> Bitwise OR18/29
  Data Type Conversion7/1 -> Bit Shift7/1
  Demux/10 -> Data Type Conversion2/1
  Data Type Conversion20/1 -> Bit Shift19/1
  Demux/21 -> Data Type Conversion17/1
  Data Type Conversion40/1 -> Bit Shift31/1
  Data Type Conversion11/1 -> Bit Shift14/1
  Data Type Conversion8/1 -> Bit Shift8/1
  Bit Shift20/1 -> Bitwise OR18/28
  Data Type Conversion38/1 -> Bit Shift29/1
  Bit Shift9/1 -> Bitwise OR18/25
  Data Type Conversion24/1 -> Bit Shift24/1
  Bit Shift19/1 -> Bitwise OR18/24
  Data Type Conversion17/1 -> Bit Shift16/1
  Demux/23 -> Data Type Conversion19/1
  Data Type Conversion16/1 -> Bit Shift20/1
  Bit Shift16/1 -> Bitwise OR18/21
  Bit Shift33/1 -> Bitwise OR18/7
  Demux/22 -> Data Type Conversion18/1
  Bit Shift30/1 -> Bitwise OR18/4
  Demux/32 -> Data Type Conversion24/1
  Data Type Conversion1/1 -> Bit Shift1/1
  Data Type Conversion19/1 -> Bit Shift18/1
  Demux/20 -> Data Type Conversion15/1
  Data Type Conversion18/1 -> Bit Shift17/1
  Data Type Conversion15/1 -> Bit Shift15/1
  Data Type Conversion37/1 -> Bit Shift28/1
  Demux/2 -> Data Type Conversion37/1
  Bit Shift17/1 -> Bitwise OR18/22
  Bit Shift3/1 -> Bitwise OR18/11
  Demux/13 -> Data Type Conversion5/1
  Data Type Conversion13/1 -> Bit Shift12/1
  Bit Shift6/1 -> Bitwise OR18/14
  Demux/30 -> Data Type Conversion22/1
  Demux/5 -> Data Type Conversion40/1
  Data Type Conversion39/1 -> Bit Shift30/1
  Demux/27 -> Data Type Conversion11/1
  Demux/8 -> Data Type Conversion43/1
  Demux/25 -> Data Type Conversion9/1
  Demux/9 -> Data Type Conversion1/1
  Data Type Conversion36/1 -> Bit Shift27/1
  Bit Shift15/1 -> Bitwise OR18/20
  Data Type Conversion2/1 -> Bit Shift2/1
  Demux/29 -> Data Type Conversion21/1
  Demux/7 -> Data Type Conversion42/1
  Data Type Conversion6/1 -> Bit Shift6/1
  Demux/11 -> Data Type Conversion3/1
  Bit Shift7/1 -> Bitwise OR18/15
  Demux/19 -> Data Type Conversion14/1
  Bit Shift34/1 -> Bitwise OR18/8
  Demux/14 -> Data Type Conversion6/1
  Demux/3 -> Data Type Conversion38/1
  Bit Shift4/1 -> Bitwise OR18/12
  Bit Shift8/1 -> Bitwise OR18/16
  Bit Shift27/1 -> Bitwise OR18/1
  Demux/24 -> Data Type Conversion20/1
  Demux/26 -> Data Type Conversion10/1
  Demux/18 -> Data Type Conversion13/1
  Data Type Conversion3/1 -> Bit Shift3/1
  DTCArray_DetectChange/1 -> Demux/1
  Bit Shift11/1 -> Bitwise OR18/17
  Bit Shift10/1 -> Bitwise OR18/26
  Bitwise OR18/1 -> DTCHeader/1

== system FVT_lib/hal/DTC_ID_and_Info ==
  DTCID : Inport
  DTC_Info : Inport  Port=2
  Bit Shift37 : hdlsllib/Logic and Bit Operations/Bit Shift  mode=Shift Left Logical  N=8
  Bitwise OR20 : simulink/Logic and Bit Operations/Bitwise Operator  logicop=OR  UseBitMask=off  NumInputPorts=2  BitMask=bin2dec('11011001')  BitMaskRealWorld=Stored Integer
  DTCID+Status : Outport
  wires:
  Bitwise OR20/1 -> DTCID+Status/1
  DTC_Info/1 -> Bitwise OR20/2  "Status"
  DTCID/1 -> Bit Shift37/1
  Bit Shift37/1 -> Bitwise OR20/1

== system FVT_lib/hal/GetCharSignal ==
  In1 : Inport
  sfcnSIL_HelpGetCSigWrap : S-Function  FunctionName=sfcnSIL_HelpGetCSigWrap  Parameters=SParameter1, SParameter2  SFunctionDeploymentMode=off  EnableBusSupport=off  mask{SParameter1=CC1-1, SParameter2=CC2}
      mask prompts: SParameter1 "P1:"; SParameter2 "P2:"
      mask Display: fprintf('Level-2 S-Function SIL_HelpGetCSig');
  Out1 : Outport
  wires:
  In1/1 -> sfcnSIL_HelpGetCSigWrap/1
  sfcnSIL_HelpGetCSigWrap/1 -> Out1/1

== system FVT_lib/hal/GetLongSignal ==
  Inport : Inport
  C Caller : CCaller  FunctionName=SIL_HelpGetLSig  PortSpecificationStruct="%)30     .    ^ 8   8    (     @         %    \"     0    !     0         %  0 \"0    $    _    07)G3F%M90  4&]R=$YA;64 4V-O<&4     26YD97@     5'EP90      4VEZ90      27-';&]B86P   X    P    !@    @    $          4    (     0    ,    !         !   P!O=70 #@   #     &    \"     0         !0    @    !     P    $         $  # &]U=  .    .     8    (    !          %    \"     $    &     0         0   ...(+2020 chars)"
  Constant1 : Constant  Value=msb
  Constant2 : Constant  Value=len
  Data Type Conversion1 : DataTypeConversion
  Data Type Conversion2 : DataTypeConversion
  val : Outport
  wires:
  Constant2/1 -> Data Type Conversion2/1
  C Caller/1 -> val/1
  Constant1/1 -> Data Type Conversion1/1
  Data Type Conversion1/1 -> C Caller/2
  Data Type Conversion2/1 -> C Caller/3
  Inport/1 -> C Caller/1

== system FVT_lib/hal/GetShortSignal ==
  In1 : Inport
  sfcnSIL_HelpGetSSigWrap : S-Function  FunctionName=sfcnSIL_HelpGetSSigWrap  Parameters=SParameter1, SParameter2  SFunctionDeploymentMode=off  EnableBusSupport=off  mask{SParameter1=CC1-1, SParameter2=CC2}
      mask prompts: SParameter1 "P1:"; SParameter2 "P2:"
      mask Display: fprintf('Level-2 S-Function SIL_HelpGetSSig');
  Out1 : Outport
  wires:
  In1/1 -> sfcnSIL_HelpGetSSigWrap/1
  sfcnSIL_HelpGetSSigWrap/1 -> Out1/1

== system FVT_lib/hal/LINReceiver ==
  Constant6 : Constant  Value=busId
  Constant7 : Constant  Value=LINArray
  Constant8 : Constant  Value=msgId
  Constant9 : Constant  Value=dlc
  Data Type Conversion{1,16,18..19} (4 alike) : DataTypeConversion  OutDataTypeStr=uint8
  Demux : Demux  Outputs=8
  LINReceive : CCaller  FunctionName=LINReceive  PortSpecificationStruct="%)30     .    X @   8    (     @         %    \"     4    !     0         %  0 \"0    $    _    07)G3F%M90  4&]R=$YA;64 4V-O<&4     26YD97@     5'EP90      4VEZ90      27-';&]B86P   X    P    !@    @    $          4    (     0    ,    !         !   P!O=70 #@   #     &    \"     0         !0    @    !     P    $         $  # &]U=  .    .     8    (    !          %    \"     $    &     0         0   ...(+2675 chars)"
  Rollcnt : Outport
  wires:
  LINReceive/1 -> Rollcnt/1
  LINReceive/2 -> [RxData]
  [RxData] -> Demux/1
  Constant7/1 -> Data Type Conversion19/1
  Data Type Conversion18/1 -> LINReceive/4
  Data Type Conversion16/1 -> LINReceive/1
  Data Type Conversion1/1 -> LINReceive/2
  Constant9/1 -> Data Type Conversion18/1
  Constant6/1 -> Data Type Conversion16/1
  Constant8/1 -> Data Type Conversion1/1
  Data Type Conversion19/1 -> LINReceive/3

== system FVT_lib/hal/LINTransmit ==
  RawData : Inport
  C Caller : CCaller  FunctionName=LINTransmit  PortSpecificationStruct="%)30     .    * <   8    (     @         %    \"     0    !     0         %  0 \"0    $    _    07)G3F%M90  4&]R=$YA;64 4V-O<&4     26YD97@     5'EP90      4VEZ90      27-';&]B86P   X    X    !@    @    $          4    (     0    4    !         !     %    8G5S260    .    .     8    (    !          %    \"     $    %     0         0    !0   &)U<TED    #@   #@    &    \"     0         !0    @    !   ...(+2086 chars)"
  Constant1 : Constant  Value=busId
  Constant2 : Constant  Value=msgId
  Constant3 : Constant  Value=dlc
  Data Type Conversion2 : DataTypeConversion  OutDataTypeStr=uint8
  Data Type Conversion3 : DataTypeConversion  OutDataTypeStr=uint8
  Data Type Conversion4 : DataTypeConversion  OutDataTypeStr=uint8
  wires:
  RawData/1 -> C Caller/3
  Constant1/1 -> Data Type Conversion3/1
  Constant2/1 -> Data Type Conversion2/1
  Data Type Conversion3/1 -> C Caller/1
  Data Type Conversion2/1 -> C Caller/2
  Constant3/1 -> Data Type Conversion4/1
  Data Type Conversion4/1 -> C Caller/4
